simulink model "arctgSensorless"  (R2024b)
settings: Solver=ode3  StartTime=0.0  StopTime=0.1  FixedStep=2e-7  RelTol=1e-3
InitFcn:
  | Pn=4;
  | Ls=8.5e-3;
  | Rs=2.875;
  | fai=0.175;
  | J=0.001;
  | Udc=311;
  | Ts=2e-7;
libraries: slpidlib x3, spsDCVoltageSourceLib x1, spsGroundLib x1, spsPermanentMagnetSynchronousMachineLib x1, simulink x1, spsThreePhaseVIMeasurementLib x1, spsUniversalBridgeLib x1, sps_lib x1
settings Model: Creator=23954  LastModifiedBy=23954

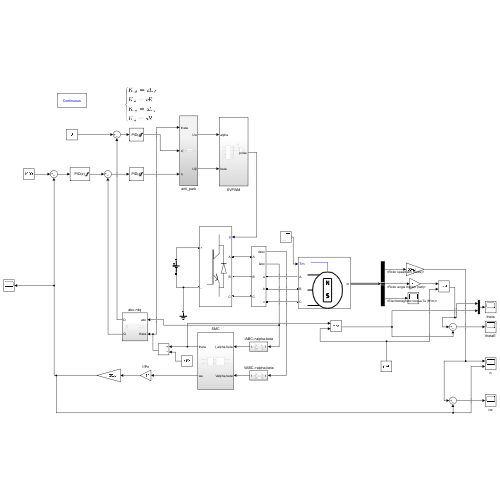
[thumbnail: Simulink's stored preview of the top-level diagram]
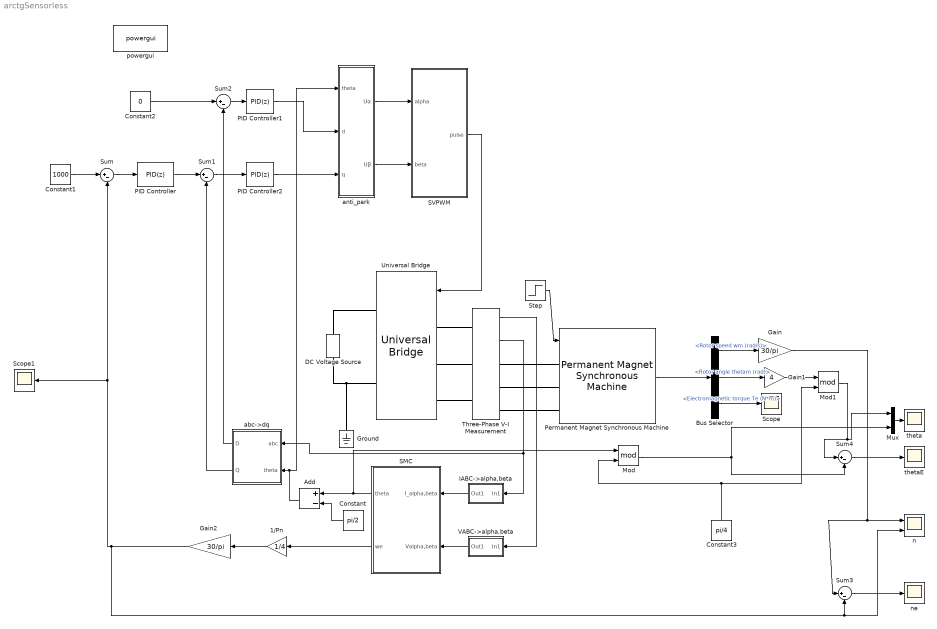
== system arctgSensorless ==
  1/Pn : Gain  Gain=1/4
  Add : Sum  Inputs=+-
  Bus Selector : BusSelector  OutputSignals=Rotor speed wm (rad/s),Rotor angle thetam (rad),Electromagnetic torque Te (N*m)
  Constant : Constant  Value=pi/2
  Constant1 : Constant  Value=1000
  Constant2 : Constant  Value=0
  Constant3 : Constant  Value=pi/4
  DC Voltage Source : spsDCVoltageSourceLib/DC Voltage Source  Amplitude=311  Measurements=None
  Gain : Gain  Gain=30/pi
  Gain1 : Gain  Gain=4
  Gain2 : Gain  Gain=30/pi
  Ground : spsGroundLib/Ground  LConnTagsString=a
  IABC->alpha,beta : Subsystem
  Mod : Math  Operator=mod
  Mod1 : Math  Operator=mod
  Mux : Mux  Inputs=2
  PID Controller : slpidlib/PID Controller  Controller=PID  Form=Parallel  TimeDomain=Discrete-time  UseExternalTs=off  SampleTime=Ts  IntegratorMethod=Forward Euler  FilterMethod=Forward Euler  ControllerParametersSource=internal  P=1  I=0.2  UseKiTs=off  D=0  UseExternalDerivativeSource=off  N=100  UseFilter=off  TunerSelectOption=Transfer Function Based (PID Tuner App)  InitialConditionSource=internal  InitialConditionForIntegrator=0  InitialConditionForFilter=0  DifferentiatorICPrevScaledInput=0  ExternalReset=none  TrackingMode=off  Kt=1  LimitOutput=on  SatLimitsSource=internal  UpperSaturationLimit=21  LowerSaturationLimit=-21  LinearizeAsGain=on  AntiWindupMode=none  Kb=1  LimitIntegrator=off  UpperIntegratorSaturationLimit=inf  LowerIntegratorSaturationLimit=-inf  POutMin=[]  POutMax=[]  IOutMin=[]  IOutMax=[]  DOutMin=[]  DOutMax=[]  NOutMin=[]  NOutMax=[]  SumOutMin=[]  SumOutMax=[]  SaturationOutMin=[]  SaturationOutMax=[]  PParamMin=[]  PParamMax=[]  IParamMin=[]  IParamMax=[]  DParamMin=[]  DParamMax=[]  NParamMin=[]  NParamMax=[]  KbParamMin=[]  KbParamMax=[]  KtParamMin=[]  KtParamMax=[]  KbOutMin=[]  KbOutMax=[]  KtOutMin=[]  KtOutMax=[]  IntegratorOutMin=[]  IntegratorOutMax=[]  FilterOutMin=[]  FilterOutMax=[]  SumI1OutMin=[]  SumI1OutMax=[]  SumI2OutMin=[]  SumI2OutMax=[]  SumI3OutMin=[]  SumI3OutMax=[]  SumI4OutMin=[]  SumI4OutMax=[]  SumDOutMin=[]  SumDOutMax=[]  DifferentiatorOutMin=[]  DifferentiatorOutMax=[]  FilterDiffOutCoefMin=[]  FilterDiffOutCoefMax=[]  ReciprocalOutMin=[]  ReciprocalOutMax=[]  SumDenOutMin=[]  SumDenOutMax=[]  SumNumOutMin=[]  SumNumOutMax=[]  DivideOutMin=[]  DivideOutMax=[]  UdiffTsProdOutMin=[]  UdiffTsProdOutMax=[]  NTsProdOutMin=[]  NTsProdOutMax=[]  UintegralTsProdOutMin=[]  UintegralTsProdOutMax=[]  UngainTsProdOutMin=[]  UngainTsProdOutMax=[]  ClampingZeroOutDataTypeStr=Inherit: Inherit via back propagation  ClampingZeroOutMin=[]  ClampingZeroOutMax=[]  FilterDenConstantOutDataTypeStr=Inherit: Inherit via back propagation  FilterDenConstantOutMin=[]  FilterDenConstantOutMax=[]  PCopyOutDataTypeStr=Inherit: Inherit via back propagation  PCopyOutMin=[]  PCopyOutMax=[]  NCopyOutDataTypeStr=Inherit: Inherit via back propagation  NCopyOutMin=[]  NCopyOutMax=[]  IntegratorContinuousStateAttributes=''  IntegratorStateMustResolveToSignalObject=off  IntegratorRTWStateStorageClass=Auto  FilterContinuousStateAttributes=''  FilterStateMustResolveToSignalObject=off  FilterRTWStateStorageClass=Auto  ParallelPVariant=InternalParameters  IdealPVariant=Disabled  IVariant=InternalParameters  DVariant=InternalParameters  IntegratorVariant=Discrete  SatVariant=Enabled  AWVariant=Passthrough  PCopyVariant=Disabled  TRVariant=Disabled  FdbkBlocksVariant=Forward  IdealPFdbkVariant=Disabled  SatFdbkVariant=Disabled  DerivativeFilterVariant=Differentiator  NVariant=Passthrough  NCopyVariant=Disabled_SignalSpec  FilterICVariant=InternalICsDifferentiator  IntegratorICVariant=InternalICs  ExternalResetVariant=Disabled  TRSumVariant=Passthrough  SumFdbkVariant=Disabled  SumVariant=Sum_PID  TsampFilterVariant=InternalTs  TsampNgainVariant=Passthrough  TsampIntegralVariant=Disabled_SignalSpec  ExternalSaturationOutDataTypeStr=Inherit: Same as second input  DerivativeSourceVariant=ErrorSignal  PreIntVariant=InternalPreInt
  PID Controller1 : slpidlib/PID Controller  Controller=PID  Form=Parallel  TimeDomain=Discrete-time  UseExternalTs=off  SampleTime=Ts  IntegratorMethod=Forward Euler  FilterMethod=Forward Euler  ControllerParametersSource=internal  P=Ls*2000  I=Rs*2000  UseKiTs=off  D=0  UseExternalDerivativeSource=off  N=100  UseFilter=off  TunerSelectOption=Transfer Function Based (PID Tuner App)  InitialConditionSource=internal  InitialConditionForIntegrator=0  InitialConditionForFilter=0  DifferentiatorICPrevScaledInput=0  ExternalReset=none  TrackingMode=off  Kt=1  LimitOutput=on  SatLimitsSource=internal  UpperSaturationLimit=350  LowerSaturationLimit=-350  LinearizeAsGain=on  AntiWindupMode=none  Kb=1  LimitIntegrator=off  UpperIntegratorSaturationLimit=inf  LowerIntegratorSaturationLimit=-inf  POutMin=[]  POutMax=[]  IOutMin=[]  IOutMax=[]  DOutMin=[]  DOutMax=[]  NOutMin=[]  NOutMax=[]  SumOutMin=[]  SumOutMax=[]  SaturationOutMin=[]  SaturationOutMax=[]  PParamMin=[]  PParamMax=[]  IParamMin=[]  IParamMax=[]  DParamMin=[]  DParamMax=[]  NParamMin=[]  NParamMax=[]  KbParamMin=[]  KbParamMax=[]  KtParamMin=[]  KtParamMax=[]  KbOutMin=[]  KbOutMax=[]  KtOutMin=[]  KtOutMax=[]  IntegratorOutMin=[]  IntegratorOutMax=[]  FilterOutMin=[]  FilterOutMax=[]  SumI1OutMin=[]  SumI1OutMax=[]  SumI2OutMin=[]  SumI2OutMax=[]  SumI3OutMin=[]  SumI3OutMax=[]  SumI4OutMin=[]  SumI4OutMax=[]  SumDOutMin=[]  SumDOutMax=[]  DifferentiatorOutMin=[]  DifferentiatorOutMax=[]  FilterDiffOutCoefMin=[]  FilterDiffOutCoefMax=[]  ReciprocalOutMin=[]  ReciprocalOutMax=[]  SumDenOutMin=[]  SumDenOutMax=[]  SumNumOutMin=[]  SumNumOutMax=[]  DivideOutMin=[]  DivideOutMax=[]  UdiffTsProdOutMin=[]  UdiffTsProdOutMax=[]  NTsProdOutMin=[]  NTsProdOutMax=[]  UintegralTsProdOutMin=[]  UintegralTsProdOutMax=[]  UngainTsProdOutMin=[]  UngainTsProdOutMax=[]  ClampingZeroOutDataTypeStr=Inherit: Inherit via back propagation  ClampingZeroOutMin=[]  ClampingZeroOutMax=[]  FilterDenConstantOutDataTypeStr=Inherit: Inherit via back propagation  FilterDenConstantOutMin=[]  FilterDenConstantOutMax=[]  PCopyOutDataTypeStr=Inherit: Inherit via back propagation  PCopyOutMin=[]  PCopyOutMax=[]  NCopyOutDataTypeStr=Inherit: Inherit via back propagation  NCopyOutMin=[]  NCopyOutMax=[]  IntegratorContinuousStateAttributes=''  IntegratorStateMustResolveToSignalObject=off  IntegratorRTWStateStorageClass=Auto  FilterContinuousStateAttributes=''  FilterStateMustResolveToSignalObject=off  FilterRTWStateStorageClass=Auto  ParallelPVariant=InternalParameters  IdealPVariant=Disabled  IVariant=InternalParameters  DVariant=InternalParameters  IntegratorVariant=Discrete  SatVariant=Enabled  AWVariant=Passthrough  PCopyVariant=Disabled  TRVariant=Disabled  FdbkBlocksVariant=Forward  IdealPFdbkVariant=Disabled  SatFdbkVariant=Disabled  DerivativeFilterVariant=Differentiator  NVariant=Passthrough  NCopyVariant=Disabled_SignalSpec  FilterICVariant=InternalICsDifferentiator  IntegratorICVariant=InternalICs  ExternalResetVariant=Disabled  TRSumVariant=Passthrough  SumFdbkVariant=Disabled  SumVariant=Sum_PID  TsampFilterVariant=InternalTs  TsampNgainVariant=Passthrough  TsampIntegralVariant=Disabled_SignalSpec  ExternalSaturationOutDataTypeStr=Inherit: Same as second input  DerivativeSourceVariant=ErrorSignal  PreIntVariant=InternalPreInt
  PID Controller2 : slpidlib/PID Controller  Controller=PID  Form=Parallel  TimeDomain=Discrete-time  UseExternalTs=off  SampleTime=Ts  IntegratorMethod=Forward Euler  FilterMethod=Forward Euler  ControllerParametersSource=internal  P=Ls*2000  I=Rs*2000  UseKiTs=off  D=0  UseExternalDerivativeSource=off  N=100  UseFilter=off  TunerSelectOption=Transfer Function Based (PID Tuner App)  InitialConditionSource=internal  InitialConditionForIntegrator=0  InitialConditionForFilter=0  DifferentiatorICPrevScaledInput=0  ExternalReset=none  TrackingMode=off  Kt=1  LimitOutput=on  SatLimitsSource=internal  UpperSaturationLimit=350  LowerSaturationLimit=-350  LinearizeAsGain=on  AntiWindupMode=none  Kb=1  LimitIntegrator=off  UpperIntegratorSaturationLimit=inf  LowerIntegratorSaturationLimit=-inf  POutMin=[]  POutMax=[]  IOutMin=[]  IOutMax=[]  DOutMin=[]  DOutMax=[]  NOutMin=[]  NOutMax=[]  SumOutMin=[]  SumOutMax=[]  SaturationOutMin=[]  SaturationOutMax=[]  PParamMin=[]  PParamMax=[]  IParamMin=[]  IParamMax=[]  DParamMin=[]  DParamMax=[]  NParamMin=[]  NParamMax=[]  KbParamMin=[]  KbParamMax=[]  KtParamMin=[]  KtParamMax=[]  KbOutMin=[]  KbOutMax=[]  KtOutMin=[]  KtOutMax=[]  IntegratorOutMin=[]  IntegratorOutMax=[]  FilterOutMin=[]  FilterOutMax=[]  SumI1OutMin=[]  SumI1OutMax=[]  SumI2OutMin=[]  SumI2OutMax=[]  SumI3OutMin=[]  SumI3OutMax=[]  SumI4OutMin=[]  SumI4OutMax=[]  SumDOutMin=[]  SumDOutMax=[]  DifferentiatorOutMin=[]  DifferentiatorOutMax=[]  FilterDiffOutCoefMin=[]  FilterDiffOutCoefMax=[]  ReciprocalOutMin=[]  ReciprocalOutMax=[]  SumDenOutMin=[]  SumDenOutMax=[]  SumNumOutMin=[]  SumNumOutMax=[]  DivideOutMin=[]  DivideOutMax=[]  UdiffTsProdOutMin=[]  UdiffTsProdOutMax=[]  NTsProdOutMin=[]  NTsProdOutMax=[]  UintegralTsProdOutMin=[]  UintegralTsProdOutMax=[]  UngainTsProdOutMin=[]  UngainTsProdOutMax=[]  ClampingZeroOutDataTypeStr=Inherit: Inherit via back propagation  ClampingZeroOutMin=[]  ClampingZeroOutMax=[]  FilterDenConstantOutDataTypeStr=Inherit: Inherit via back propagation  FilterDenConstantOutMin=[]  FilterDenConstantOutMax=[]  PCopyOutDataTypeStr=Inherit: Inherit via back propagation  PCopyOutMin=[]  PCopyOutMax=[]  NCopyOutDataTypeStr=Inherit: Inherit via back propagation  NCopyOutMin=[]  NCopyOutMax=[]  IntegratorContinuousStateAttributes=''  IntegratorStateMustResolveToSignalObject=off  IntegratorRTWStateStorageClass=Auto  FilterContinuousStateAttributes=''  FilterStateMustResolveToSignalObject=off  FilterRTWStateStorageClass=Auto  ParallelPVariant=InternalParameters  IdealPVariant=Disabled  IVariant=InternalParameters  DVariant=InternalParameters  IntegratorVariant=Discrete  SatVariant=Enabled  AWVariant=Passthrough  PCopyVariant=Disabled  TRVariant=Disabled  FdbkBlocksVariant=Forward  IdealPFdbkVariant=Disabled  SatFdbkVariant=Disabled  DerivativeFilterVariant=Differentiator  NVariant=Passthrough  NCopyVariant=Disabled_SignalSpec  FilterICVariant=InternalICsDifferentiator  IntegratorICVariant=InternalICs  ExternalResetVariant=Disabled  TRSumVariant=Passthrough  SumFdbkVariant=Disabled  SumVariant=Sum_PID  TsampFilterVariant=InternalTs  TsampNgainVariant=Passthrough  TsampIntegralVariant=Disabled_SignalSpec  ExternalSaturationOutDataTypeStr=Inherit: Same as second input  DerivativeSourceVariant=ErrorSignal  PreIntVariant=InternalPreInt
  Permanent Magnet Synchronous Machine : spsPermanentMagnetSynchronousMachineLib/Permanent Magnet Synchronous Machine  NbPhases=3  FluxDistribution=Sinusoidal  RotorType=Salient-pole  MechanicalLoad=Torque Tm  PresetModel=No  ShowDetailedParameters=on  MeasurementBus=off  Resistance=2.875  Inductance=8.5e-3  dqInductances=[8.5e-3,8.5e-3]  La=0.0085  MachineConstant=Flux linkage established by magnets (V.s)  Flux=0.175  VoltageCst=126.966  TorqueCst=1.05  Flat=120  Mechanical=[0.001 ,0 ,4]  PolePairs=4  InitialConditions=[0,0, 0,0]  InitialConditions5ph=[0 0 0 0 0 0]  RefAngle=90 degrees behind phase A axis (modified Park)  IterativeDiscreteModel=Trapezoidal non iterative  TsBlock=-1  TsPowergui=0
  SMC : Subsystem
  SVPWM : Subsystem
  Scope : Scope
  Scope1 : Scope
  Step : Step  Time=0.05  After=20  SampleTime=0
  Sum{,1..4} (5 alike) : Sum  Inputs=|+-
  Three-Phase V-I Measurement : spsThreePhaseVIMeasurementLib/Three-Phase V-I Measurement  VoltageMeasurement=phase-to-ground  SetLabelV=off  LabelV=Vabc  Vpu=off  VpuLL=off  CurrentMeasurement=yes  SetLabelI=off  LabelI=Iabc  Ipu=off  Pbase=100e6  Vbase=500e3  OutputType=Complex  PhasorSimulation=off  PSBequivalent=0
  Universal Bridge : spsUniversalBridgeLib/Universal Bridge  Arms=3  SnubberResistance=1e5  SnubberCapacitance=inf  Device=IGBT / Diodes  Ron=1e-3  Lon=0  ForwardVoltages="[  0  0  ]"  ForwardVoltage=0  GTOparameters=[ 10e-6 , 20e-6 ]  IGBTparameters=[ 1e-6 , 2e-6 ]  Measurements=None  Measurements_2=None  converterType=Rectifier
  VABC->alpha,beta : Subsystem
  abc->dq : Subsystem
  anti_park : Subsystem
  n : Scope  NumInputPorts=2
  ne : Scope
  powergui : sps_lib/powergui  Priority=1  SimulationMode=Continuous  SampleTime=50e-6  frequency=60  Iterations=50  frequencyindice=0  Pbase=100e6  ErrMax=1e-4  UnitsV=kV  UnitsW=MW  buscounter=0  FunctionMessages=off  echomessages=off  EnableUseOfTLC=off  CurrentSourceSwitches=off  DisableSnubberDevices=off  DisableRonSwitches=off  DisableVfSwitches=off  DisplayEquations=off  AutomaticDiscreteSolvers=off  SolverType=Tustin/Backward Euler (TBE)  Interpol=off  ExternalGateDelay=off  methode=off  Ts=100  x0status=blocks  SPID=on  SwTol=0  HookPort=off  NonlinearTolerance=1e-4  nMaxIteration=100  ContinueOnMaxIteration=off  RestoreLinks=warning  ResistiveCurrentMeasurement=off  Frange=[0:2:500]  Ylog=off  Xlog=on  ShowGrid=off  save=off  variable=ZData  structure=0  ZoomFFT=off  StartTime=0.0  cycles=1  DisplayStyle=1  fundamental=60  FreqAxis=off  MaxFrequency=1000  frequencyindicesteady=1  RmsSteady=1  display=off
  theta : Scope
  thetaE : Scope
  wires:
  Step/1 -> Permanent Magnet Synchronous Machine/1
  Permanent Magnet Synchronous Machine/1 -> Bus Selector/1
  Bus Selector/1 -> Gain/1  "<Rotor speed wm (rad/s)>"
  Bus Selector/2 -> Gain1/1  "<Rotor angle thetam (rad)>"
  Bus Selector/3 -> Scope/1  "<Electromagnetic torque Te (N*m)>"
  Three-Phase V-I Measurement/2 -> IABC->alpha,beta/1(In1), abc->dq/1(abc)
  Three-Phase V-I Measurement/1 -> VABC->alpha,beta/1(In1)
  IABC->alpha,beta/1(Out1) -> SMC/1(I_alpha,beta)
  VABC->alpha,beta/1(Out1) -> SMC/2(Valpha,beta)
  Constant/1 -> Add/2
  Constant1/1 -> Sum/1
  Gain2/1 -> n/2, Sum3/2, Sum/2, Scope1/1
  Add/1 -> anti_park/1(theta), abc->dq/2(theta)
  Sum/1 -> PID Controller/1
  PID Controller/1 -> Sum1/1
  abc->dq/2(Q) -> Sum1/2
  abc->dq/1(D) -> Sum2/2
  Constant2/1 -> Sum2/1
  Sum2/1 -> PID Controller1/1
  Sum1/1 -> PID Controller2/1
  anti_park/2(Uβ) -> SVPWM/2(beta)
  anti_park/1(Uα) -> SVPWM/1(alpha)
  PID Controller1/1 -> anti_park/2(d)
  PID Controller2/1 -> anti_park/3(q)
  SVPWM/1(pulse) -> Universal Bridge/1
  Mux/1 -> theta/1
  Sum4/1 -> thetaE/1
  Gain/1 -> n/1, Sum3/1
  Sum3/1 -> ne/1
  SMC/1(theta) -> Mod/1, Add/1
  Mod1/1 -> Sum4/1, Mux/1
  1/Pn/1 -> Gain2/1
  SMC/2(we) -> 1/Pn/1
  Constant3/1 -> Mod/2, Mod1/2
  Mod/1 -> Mux/2, Sum4/2
  Gain1/1 -> Mod1/1
  connections:
  DC Voltage Source/RConn1 -- Universal Bridge/RConn1
  DC Voltage Source/LConn1 -- Ground/LConn1 -- Universal Bridge/RConn2
  Three-Phase V-I Measurement/LConn1 -- Universal Bridge/LConn1
  Universal Bridge/LConn2 -- Three-Phase V-I Measurement/LConn2
  Universal Bridge/LConn3 -- Three-Phase V-I Measurement/LConn3
  Three-Phase V-I Measurement/RConn1 -- Permanent Magnet Synchronous Machine/LConn1
  Three-Phase V-I Measurement/RConn2 -- Permanent Magnet Synchronous Machine/LConn2
  Three-Phase V-I Measurement/RConn3 -- Permanent Magnet Synchronous Machine/LConn3

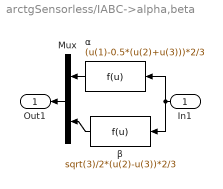
== system arctgSensorless/IABC->alpha,beta ==
  In1 : Inport
  Mux : Mux  Inputs=2
  α : Fcn  Expr=(u(1)-0.5*(u(2)+u(3)))*2/3
  β : Fcn  Expr=sqrt(3)/2*(u(2)-u(3))*2/3
  Out1 : Outport
  wires:
  In1/1 -> α/1, β/1
  α/1 -> Mux/1
  β/1 -> Mux/2
  Mux/1 -> Out1/1

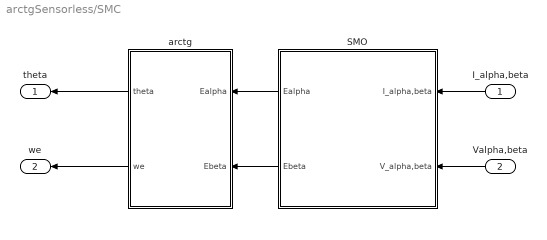
== system arctgSensorless/SMC ==
  I_alpha,beta : Inport
  Valpha,beta : Inport  Port=2
  SMO : Subsystem
  arctg : Subsystem
  theta : Outport
  we : Outport  Port=2
  wires:
  I_alpha,beta/1 -> SMO/1(I_alpha,beta)
  Valpha,beta/1 -> SMO/2(V_alpha,beta)
  SMO/1(Ealpha) -> arctg/1(Ealpha)
  SMO/2(Ebeta) -> arctg/2(Ebeta)
  arctg/1(theta) -> theta/1
  arctg/2(we) -> we/1

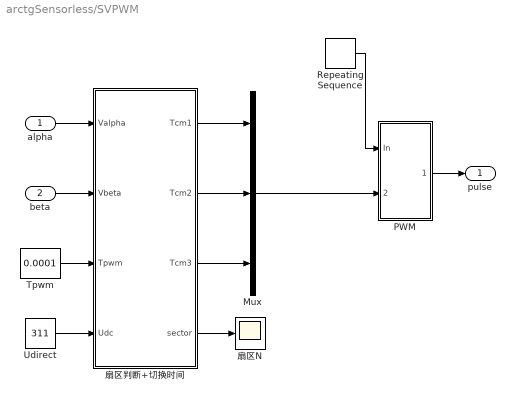
== system arctgSensorless/SVPWM ==
  alpha : Inport
  beta : Inport  Port=2
  Mux : Mux  Inputs=3
  PWM : Subsystem
  Repeating Sequence : simulink/Sources/Repeating Sequence  rep_seq_t=[0 0.00005 0.0001]  rep_seq_y=[0 0.00005 0]
  Tpwm : Constant  Value=0.0001
  Udirect : Constant  Value=311
  扇区N : Scope
  扇区判断+切换时间 : MATLAB Function  TreatAsAtomicUnit=on
  pulse : Outport
  wires:
  alpha/1 -> 扇区判断+切换时间/1(Valpha)
  beta/1 -> 扇区判断+切换时间/2(Vbeta)
  Tpwm/1 -> 扇区判断+切换时间/3(Tpwm)
  Udirect/1 -> 扇区判断+切换时间/4(Udc)
  扇区判断+切换时间/4(sector) -> 扇区N/1
  Mux/1 -> PWM/2(Tcm123)
  PWM/1(PWM) -> pulse/1
  Repeating Sequence/1 -> PWM/1(In)
  扇区判断+切换时间/2(Tcm2) -> Mux/2
  扇区判断+切换时间/1(Tcm1) -> Mux/1
  扇区判断+切换时间/3(Tcm3) -> Mux/3

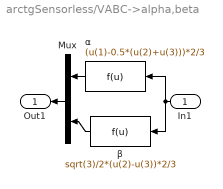
== system arctgSensorless/VABC->alpha,beta ==
  In1 : Inport
  Mux : Mux  Inputs=2
  α : Fcn  Expr=(u(1)-0.5*(u(2)+u(3)))*2/3
  β : Fcn  Expr=sqrt(3)/2*(u(2)-u(3))*2/3
  Out1 : Outport
  wires:
  In1/1 -> α/1, β/1
  α/1 -> Mux/1
  β/1 -> Mux/2
  Mux/1 -> Out1/1

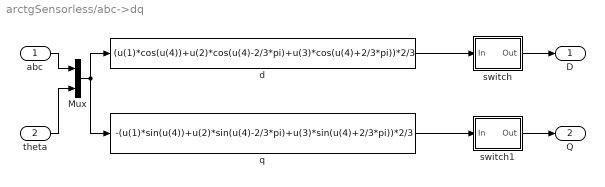
== system arctgSensorless/abc->dq ==
  abc : Inport
  theta : Inport  Port=2
  Mux : Mux  Inputs=2
  d : Fcn  Expr=(u(1)*cos(u(4))+u(2)*cos(u(4)-2/3*pi)+u(3)*cos(u(4)+2/3*pi))*2/3
  q : Fcn  Expr=-(u(1)*sin(u(4))+u(2)*sin(u(4)-2/3*pi)+u(3)*sin(u(4)+2/3*pi))*2/3
  switch : Subsystem
  switch1 : Subsystem
  D : Outport
  Q : Outport  Port=2
  wires:
  abc/1 -> Mux/1
  theta/1 -> Mux/2
  Mux/1 -> d/1, q/1
  d/1 -> switch/1(In)
  switch/1(Out) -> D/1
  q/1 -> switch1/1(In)
  switch1/1(Out) -> Q/1

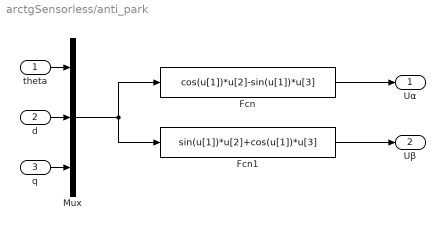
== system arctgSensorless/anti_park ==
  theta : Inport
  d : Inport  Port=2
  q : Inport  Port=3
  Fcn : Fcn  Expr=cos(u[1])*u[2]-sin(u[1])*u[3]
  Fcn1 : Fcn  Expr=sin(u[1])*u[2]+cos(u[1])*u[3]
  Mux : Mux  Inputs=3
  Uα : Outport
  Uβ : Outport  Port=2
  wires:
  Fcn/1 -> Uα/1
  Fcn1/1 -> Uβ/1
  theta/1 -> Mux/1
  Mux/1 -> Fcn1/1, Fcn/1
  d/1 -> Mux/2
  q/1 -> Mux/3

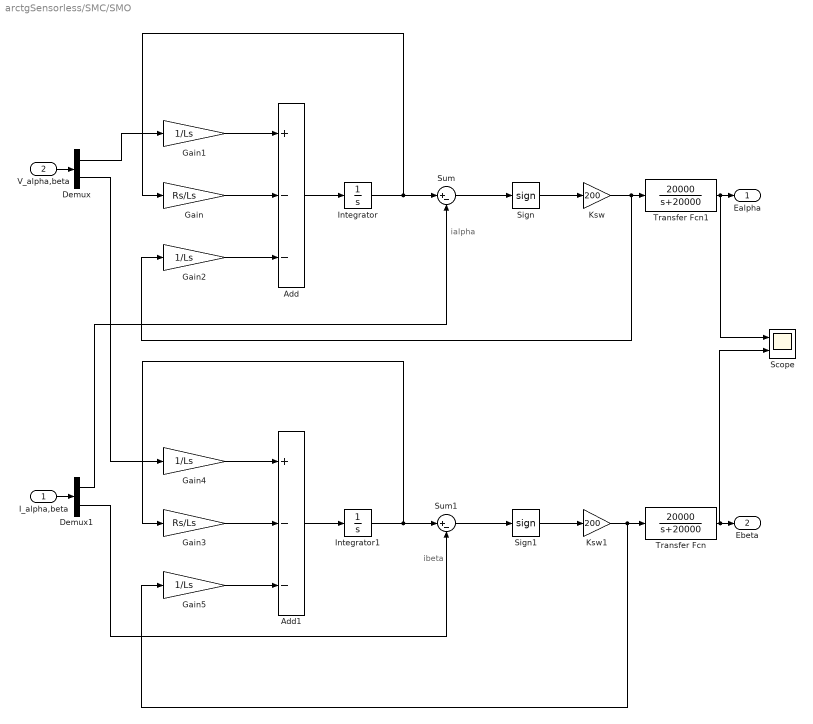
== system arctgSensorless/SMC/SMO ==
  note: ibeta
  note: ialpha
  I_alpha,beta : Inport
  V_alpha,beta : Inport  Port=2
  Add : Sum  Inputs=+--
  Add1 : Sum  Inputs=+--
  Demux : Demux  Outputs=2
  Demux1 : Demux  Outputs=2
  Gain : Gain  Gain=Rs/Ls
  Gain{1..2,4..5} (4 alike) : Gain  Gain=1/Ls
  Gain3 : Gain  Gain=Rs/Ls
  Integrator : Integrator
  Integrator1 : Integrator
  Ksw : Gain  Gain=200
  Ksw1 : Gain  Gain=200
  Scope : Scope  NumInputPorts=2
  Sign : Signum
  Sign1 : Signum
  Sum : Sum  Inputs=|+-
  Sum1 : Sum  Inputs=|+-
  Transfer Fcn : TransferFcn  Numerator=[20000]  Denominator=[1 20000]
  Transfer Fcn1 : TransferFcn  Numerator=[20000]  Denominator=[1 20000]
  Ealpha : Outport
  Ebeta : Outport  Port=2
  wires:
  V_alpha,beta/1 -> Demux/1
  Demux/1 -> Gain1/1
  Gain1/1 -> Add/1
  Gain/1 -> Add/2
  Gain2/1 -> Add/3
  Add/1 -> Integrator/1
  Integrator/1 -> Sum/1, Gain/1
  Sum/1 -> Sign/1
  Sign/1 -> Ksw/1
  Ksw/1 -> Gain2/1, Transfer Fcn1/1
  Integrator1/1 -> Sum1/1, Gain3/1
  Gain5/1 -> Add1/3
  Gain4/1 -> Add1/1
  I_alpha,beta/1 -> Demux1/1
  Add1/1 -> Integrator1/1
  Sign1/1 -> Ksw1/1
  Ksw1/1 -> Transfer Fcn/1, Gain5/1
  Sum1/1 -> Sign1/1
  Gain3/1 -> Add1/2
  Demux/2 -> Gain4/1
  Demux1/1 -> Sum/2
  Demux1/2 -> Sum1/2
  Transfer Fcn1/1 -> Scope/1, Ealpha/1
  Transfer Fcn/1 -> Scope/2, Ebeta/1

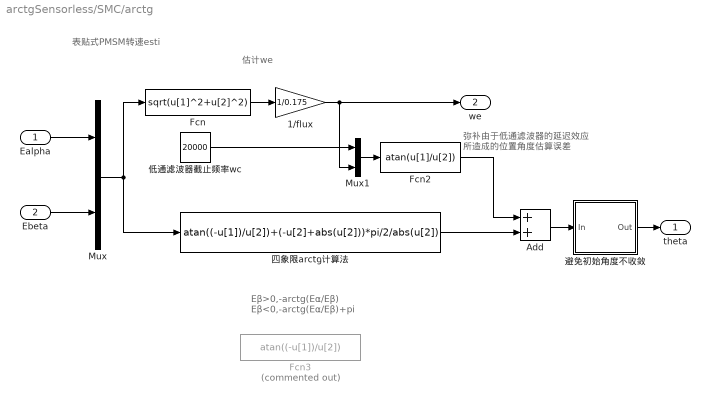
== system arctgSensorless/SMC/arctg ==
  note: Eβ>0,-arctg(Eα/Eβ)
      | Eβ<0,-arctg(Eα/Eβ)+pi
  note: 弥补由于低通滤波器的延迟效应
      | 所造成的位置角度估算误差
  note: 表贴式PMSM转速esti
  note: 估计we
  Ealpha : Inport
  Ebeta : Inport  Port=2
  1/flux : Gain  Gain=1/0.175
  Add : Sum
  Fcn : Fcn  Expr=sqrt(u[1]^2+u[2]^2)
  Fcn2 : Fcn  Expr=atan(u[1]/u[2])
  Fcn3 : Fcn  Commented=on  Expr=atan((-u[1])/u[2])
  Mux : Mux  Inputs=2
  Mux1 : Mux  Inputs=2
  低通滤波器截止频率wc : Constant  Value=20000
  四象限arctg计算法 : Fcn  Expr=atan((-u[1])/u[2])+(-u[2]+abs(u[2]))*pi/2/abs(u[2])
  避免初始角度不收敛 : Subsystem
  theta : Outport
  we : Outport  Port=2
  wires:
  Ealpha/1 -> Mux/1
  Ebeta/1 -> Mux/2
  Mux/1 -> 四象限arctg计算法/1, Fcn/1
  Fcn/1 -> 1/flux/1
  1/flux/1 -> Mux1/2, we/1
  Mux1/1 -> Fcn2/1
  Fcn2/1 -> Add/1
  Add/1 -> 避免初始角度不收敛/1(In)
  避免初始角度不收敛/1(Out) -> theta/1
  四象限arctg计算法/1 -> Add/2
  低通滤波器截止频率wc/1 -> Mux1/1

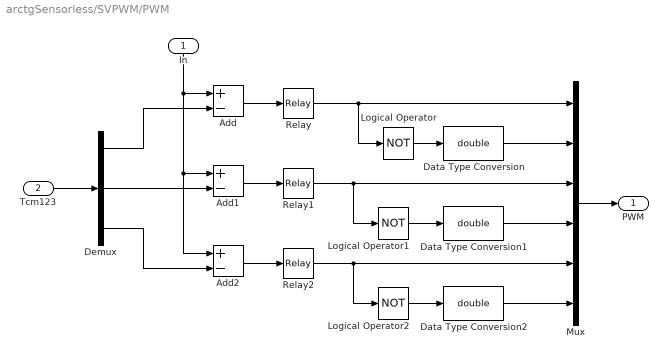
== system arctgSensorless/SVPWM/PWM ==
  In : Inport
  Tcm123 : Inport  Port=2
  Add : Sum  Inputs=+-
  Add1 : Sum  Inputs=+-
  Add2 : Sum  Inputs=+-
  Data Type Conversion : DataTypeConversion  OutDataTypeStr=double  SaturateOnIntegerOverflow=off  RndMeth=Floor
  Data Type Conversion1 : DataTypeConversion  OutDataTypeStr=double  SaturateOnIntegerOverflow=off  RndMeth=Floor
  Data Type Conversion2 : DataTypeConversion  OutDataTypeStr=double  SaturateOnIntegerOverflow=off  RndMeth=Floor
  Demux : Demux  Outputs=3
  Logical Operator : Logic  Operator=NOT  AllPortsSameDT=off  OutDataTypeStr=boolean
  Logical Operator1 : Logic  Operator=NOT  AllPortsSameDT=off  OutDataTypeStr=boolean
  Logical Operator2 : Logic  Operator=NOT  AllPortsSameDT=off  OutDataTypeStr=boolean
  Mux : Mux  Inputs=6
  Relay : Relay  OffSwitchValue=-eps
  Relay1 : Relay  OffSwitchValue=-eps
  Relay2 : Relay  OffSwitchValue=-eps
  PWM : Outport
  wires:
  Demux/3 -> Add2/2
  Demux/2 -> Add1/2
  Demux/1 -> Add/2
  Relay2/1 -> Mux/5, Logical Operator2/1
  Relay1/1 -> Mux/3, Logical Operator1/1
  Relay/1 -> Logical Operator/1, Mux/1
  Mux/1 -> PWM/1
  Data Type Conversion/1 -> Mux/2
  Data Type Conversion1/1 -> Mux/4
  Data Type Conversion2/1 -> Mux/6
  Logical Operator2/1 -> Data Type Conversion2/1
  Logical Operator1/1 -> Data Type Conversion1/1
  Logical Operator/1 -> Data Type Conversion/1
  Add1/1 -> Relay1/1
  Add2/1 -> Relay2/1
  Add/1 -> Relay/1
  In/1 -> Add/1, Add2/1, Add1/1
  Tcm123/1 -> Demux/1

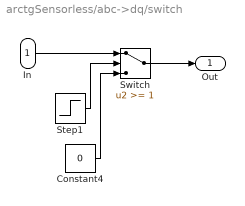
== system arctgSensorless/abc->dq/switch ==
  In : Inport
  Constant4 : Constant  Value=0
  Step1 : Step  Time=0.001  SampleTime=0
  Switch : Switch  Threshold=1  SaturateOnIntegerOverflow=off  InputSameDT=off
  Out : Outport
  wires:
  Step1/1 -> Switch/2
  Constant4/1 -> Switch/3
  In/1 -> Switch/1
  Switch/1 -> Out/1

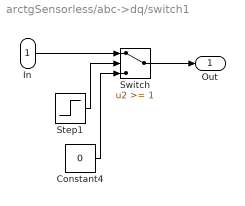
== system arctgSensorless/abc->dq/switch1 ==
  In : Inport
  Constant4 : Constant  Value=0
  Step1 : Step  Time=0.001  SampleTime=0
  Switch : Switch  Threshold=1  SaturateOnIntegerOverflow=off  InputSameDT=off
  Out : Outport
  wires:
  Step1/1 -> Switch/2
  Constant4/1 -> Switch/3
  In/1 -> Switch/1
  Switch/1 -> Out/1

== system arctgSensorless/SMC/arctg/避免初始角度不收敛 ==
  In : Inport
  Constant4 : Constant  Value=0
  Step1 : Step  Time=0.001  SampleTime=0
  Switch : Switch  Threshold=1  SaturateOnIntegerOverflow=off  InputSameDT=off
  Out : Outport
  wires:
  Step1/1 -> Switch/2
  Constant4/1 -> Switch/3
  In/1 -> Switch/1
  Switch/1 -> Out/1

== matlab function arctgSensorless/SVPWM/扇区判断+切换时间 ==
  data: Valpha input; Tcm1 output; Vbeta input; Tpwm input; Udc input; Tcm2 output; Tcm3 output; sector output
function [ Tcm1, Tcm2,  Tcm3,  sector] = fcn(Valpha, Vbeta, Tpwm, Udc)

% #codegen
%变量初始化
sector = 0;
Tcm1 = 0;
Tcm2 = 0;
Tcm3 = 0;
% = = = = = = = = Parameters statement = = = = = = = = = = = = = = = =
%P37 2-18

Vref1 = Vbeta;
Vref2 = ( sqrt(3)*Valpha- Vbeta) / 2;
Vref3 = ( -sqrt(3)*Valpha- Vbeta) / 2;
%＝= = = = = = = Sector calculation=================
%扇区判断
if  (Vref1> 0)
    sector = 1;
end
if  (Vref2> 0)
    sector = sector + 2;
end
if (Vref3> 0)
    sector = sector + 4;
end


%＝＝＝＝＝＝＝＝ X Y Z calculation===================
%P38 2-21

X = sqrt(3) * Vbeta * Tpwm/Udc;
Y = Tpwm/Udc * (3/2 *Valpha + sqrt(3)/2 * Vbeta);
Z = Tpwm/Udc * (-3/2 * Valpha + sqrt(3)/2 * Vbeta);

% = = = =======Duty ratio calculation================
%根据表2-5计算

switch (sector)
    case 1
        T1 = Z; T2 = Y;
    case 2
        T1 = Y; T2 = - X;
    case 3
        T1 = -Z; T2 = X;
    case 4
        T1 = -X; T2 = Z;
    case 5
        T1 = X; T2 = -Y;
    otherwise
        T1 = -Y; T2 = -Z;
end
%过调制处理
if T1 + T2 > Tpwm
    T1 = T1/(T1 + T2);
    T2 = T2/(T1+ T2);
else
    T1 = T1;
    T2 = T2;
end

ta= (Tpwm -(T1+T2))/ 4.0;
tb = ta+ T1/ 2;
tc = tb + T2/ 2;

%＝= = =======Duty ratio calculation================
%根据表2-6计算 各扇区时间切换点
switch (sector)
    case 1
        Tcm1 = tb;
        Tcm2 = ta;
        Tcm3 = tc;
    case 2
        Tcm1 = ta;
        Tcm2 = tc;
        Tcm3 = tb;
    case 3
        Tcm1 = ta;
        Tcm2 = tb;
        Tcm3 = tc;
    case 4
        Tcm1 = tc;
        Tcm2 = tb;
        Tcm3 = ta;
    case 5
        Tcm1 = tc;
        Tcm2 = ta;
        Tcm3 = tb;
    case 6
        Tcm1 = tb;
        Tcm2 = tc;
        Tcm3 = ta;
end
end
